simulink model "TST_InjCrv_PoI2Cor"  (R2016b)
settings: Solver=FixedStepDiscrete  StartTime=0.0  StopTime=simTime  FixedStep=sampleTime  RelTol=1e-3
values from neighbouring files (symbols this model uses):
  testCase = 1    [initTST_InjCrv_PoI2Cor_001.m]
libraries: simulink x5, UnitTest_Lib x3
settings Model: Creator=zhengjinyan  LastModifiedBy=zhengjinyan
settings DebuggingCC: SignalRangeChecking=error

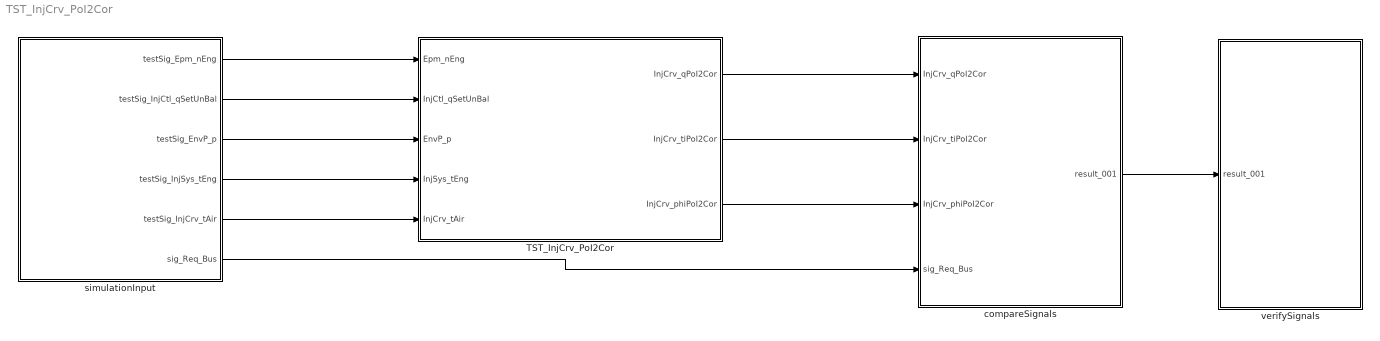
== system TST_InjCrv_PoI2Cor ==
  TST_InjCrv_PoI2Cor : Subsystem
  compareSignals : Subsystem
  simulationInput : Subsystem
  verifySignals : Subsystem
  wires:
  simulationInput/1(testSig_Epm_nEng) -> TST_InjCrv_PoI2Cor/1(Epm_nEng)
  simulationInput/2(testSig_InjCtl_qSetUnBal) -> TST_InjCrv_PoI2Cor/2(InjCtl_qSetUnBal)
  simulationInput/3(testSig_EnvP_p) -> TST_InjCrv_PoI2Cor/3(EnvP_p)
  simulationInput/4(testSig_InjSys_tEng) -> TST_InjCrv_PoI2Cor/4(InjSys_tEng)
  simulationInput/5(testSig_InjCrv_tAir) -> TST_InjCrv_PoI2Cor/5(InjCrv_tAir)
  TST_InjCrv_PoI2Cor/1(InjCrv_qPoI2Cor) -> compareSignals/1(InjCrv_qPoI2Cor)
  TST_InjCrv_PoI2Cor/2(InjCrv_tiPoI2Cor) -> compareSignals/2(InjCrv_tiPoI2Cor)
  TST_InjCrv_PoI2Cor/3(InjCrv_phiPoI2Cor) -> compareSignals/3(InjCrv_phiPoI2Cor)
  simulationInput/6(sig_Req_Bus) -> compareSignals/4(sig_Req_Bus)
  compareSignals/1(result_001) -> verifySignals/1(result_001)

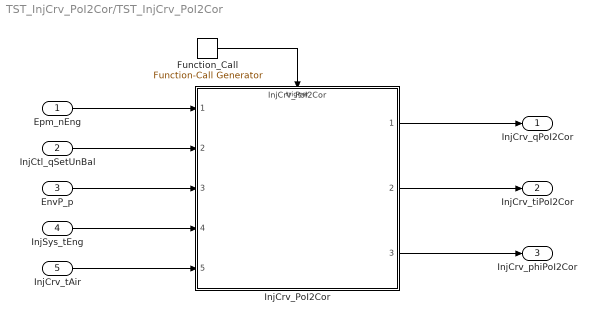
== system TST_InjCrv_PoI2Cor/TST_InjCrv_PoI2Cor ==
  Epm_nEng : Inport
  InjCtl_qSetUnBal : Inport  Port=2
  EnvP_p : Inport  Port=3
  InjSys_tEng : Inport  Port=4
  InjCrv_tAir : Inport  Port=5
  Function_Call : simulink/Ports & Subsystems/Function-Call Generator  sample_time=sampleTime  numberOfIterations=1
  InjCrv_PoI2Cor : ModelReference  ModelNameDialog=InjCrv_PoI2Cor  SimulationMode=Normal  ModelReferenceVersion=1.32  TriggerPortName=function  TriggerPortTriggerType=function-call  TriggerPortStatesWhenEnabling=held
  InjCrv_qPoI2Cor : Outport
  InjCrv_tiPoI2Cor : Outport  Port=2
  InjCrv_phiPoI2Cor : Outport  Port=3
  wires:
  Function_Call/1 -> InjCrv_PoI2Cor/Trigger
  Epm_nEng/1 -> InjCrv_PoI2Cor/1
  InjCtl_qSetUnBal/1 -> InjCrv_PoI2Cor/2
  EnvP_p/1 -> InjCrv_PoI2Cor/3
  InjSys_tEng/1 -> InjCrv_PoI2Cor/4
  InjCrv_tAir/1 -> InjCrv_PoI2Cor/5
  InjCrv_PoI2Cor/1 -> InjCrv_qPoI2Cor/1
  InjCrv_PoI2Cor/2 -> InjCrv_tiPoI2Cor/1
  InjCrv_PoI2Cor/3 -> InjCrv_phiPoI2Cor/1

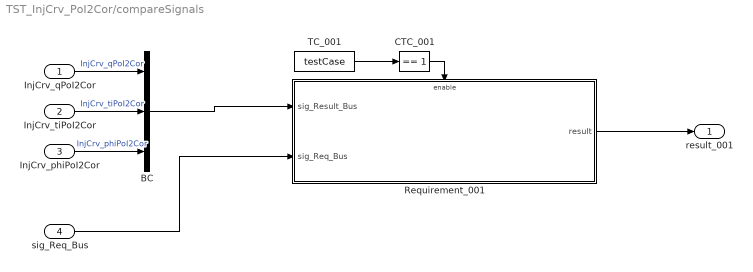
== system TST_InjCrv_PoI2Cor/compareSignals ==
  InjCrv_qPoI2Cor : Inport
  InjCrv_tiPoI2Cor : Inport  Port=2
  InjCrv_phiPoI2Cor : Inport  Port=3
  sig_Req_Bus : Inport  Port=4
  BC : BusCreator  Inputs=3
  CTC_001 : simulink/Logic and Bit Operations/Compare To Constant  relop===  const=1  OutDataTypeStr=boolean
  Requirement_001 : Subsystem
  TC_001 : Constant  Value=testCase
  result_001 : Outport
  wires:
  InjCrv_qPoI2Cor/1 -> BC/1  "InjCrv_qPoI2Cor"
  InjCrv_tiPoI2Cor/1 -> BC/2  "InjCrv_tiPoI2Cor"
  InjCrv_phiPoI2Cor/1 -> BC/3  "InjCrv_phiPoI2Cor"
  TC_001/1 -> CTC_001/1
  CTC_001/1 -> Requirement_001/Enable
  sig_Req_Bus/1 -> Requirement_001/2(sig_Req_Bus)
  BC/1 -> Requirement_001/1(sig_Result_Bus)
  Requirement_001/1(result) -> result_001/1

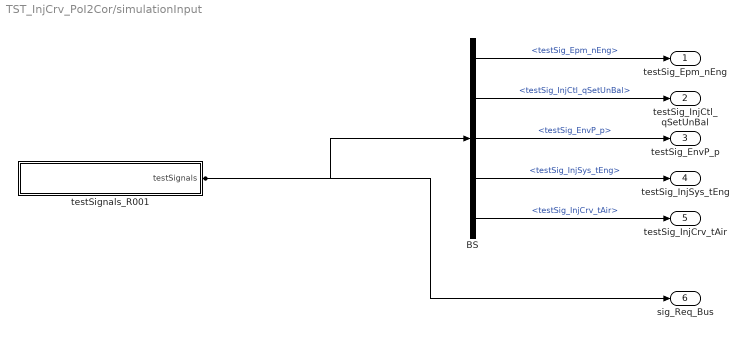
== system TST_InjCrv_PoI2Cor/simulationInput ==
  BS : BusSelector  OutputSignals=testSig_Epm_nEng,testSig_InjCtl_qSetUnBal,testSig_EnvP_p,testSig_InjSys_tEng,testSig_InjCrv_tAir
  testSignals_R001 : Subsystem
  testSig_Epm_nEng : Outport
  testSig_InjCtl_qSetUnBal : Outport  Port=2
  testSig_EnvP_p : Outport  Port=3
  testSig_InjSys_tEng : Outport  Port=4
  testSig_InjCrv_tAir : Outport  Port=5
  sig_Req_Bus : Outport  Port=6
  wires:
  BS/1 -> testSig_Epm_nEng/1  "<testSig_Epm_nEng>"
  BS/2 -> testSig_InjCtl_qSetUnBal/1  "<testSig_InjCtl_qSetUnBal>"
  BS/3 -> testSig_EnvP_p/1  "<testSig_EnvP_p>"
  BS/4 -> testSig_InjSys_tEng/1  "<testSig_InjSys_tEng>"
  BS/5 -> testSig_InjCrv_tAir/1  "<testSig_InjCrv_tAir>"
  testSignals_R001/1(testSignals) -> BS/1, sig_Req_Bus/1

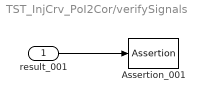
== system TST_InjCrv_PoI2Cor/verifySignals ==
  result_001 : Inport
  Assertion_001 : Assertion  Enabled=off
  wires:
  result_001/1 -> Assertion_001/1

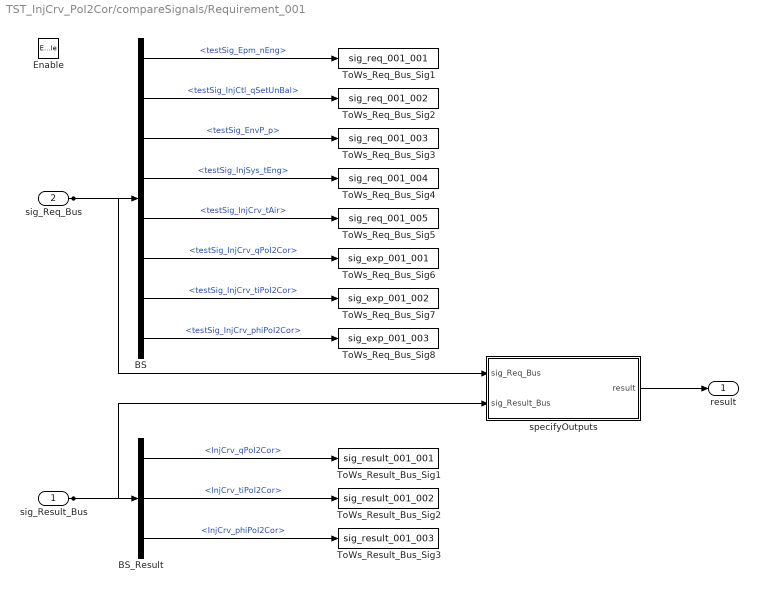
== system TST_InjCrv_PoI2Cor/compareSignals/Requirement_001 ==
  sig_Result_Bus : Inport
  sig_Req_Bus : Inport  Port=2
  Enable : EnablePort
  BS : BusSelector  OutputSignals=testSig_Epm_nEng,testSig_InjCtl_qSetUnBal,testSig_EnvP_p,testSig_InjSys_tEng,testSig_InjCrv_tAir,testSig_InjCrv_qPoI2Cor,testSig_InjCrv_tiPoI2Cor,testSig_InjCrv_phiPoI2Cor
  BS_Result : BusSelector  OutputSignals=InjCrv_qPoI2Cor,InjCrv_tiPoI2Cor,InjCrv_phiPoI2Cor
  ToWs_Req_Bus_Sig1 : ToWorkspace  VariableName=sig_req_001_001  SaveFormat=Structure With Time
  ToWs_Req_Bus_Sig2 : ToWorkspace  VariableName=sig_req_001_002  SaveFormat=Structure With Time
  ToWs_Req_Bus_Sig3 : ToWorkspace  VariableName=sig_req_001_003  SaveFormat=Structure With Time
  ToWs_Req_Bus_Sig4 : ToWorkspace  VariableName=sig_req_001_004  SaveFormat=Structure With Time
  ToWs_Req_Bus_Sig5 : ToWorkspace  VariableName=sig_req_001_005  SaveFormat=Structure With Time
  ToWs_Req_Bus_Sig6 : ToWorkspace  VariableName=sig_exp_001_001  SaveFormat=Structure With Time
  ToWs_Req_Bus_Sig7 : ToWorkspace  VariableName=sig_exp_001_002  SaveFormat=Structure With Time
  ToWs_Req_Bus_Sig8 : ToWorkspace  VariableName=sig_exp_001_003  SaveFormat=Structure With Time
  ToWs_Result_Bus_Sig1 : ToWorkspace  VariableName=sig_result_001_001  SaveFormat=Structure With Time
  ToWs_Result_Bus_Sig2 : ToWorkspace  VariableName=sig_result_001_002  SaveFormat=Structure With Time
  ToWs_Result_Bus_Sig3 : ToWorkspace  VariableName=sig_result_001_003  SaveFormat=Structure With Time
  specifyOutputs : Subsystem
  result : Outport
  wires:
  sig_Req_Bus/1 -> BS/1, specifyOutputs/1(sig_Req_Bus)
  BS/1 -> ToWs_Req_Bus_Sig1/1  "<testSig_Epm_nEng>"
  BS/2 -> ToWs_Req_Bus_Sig2/1  "<testSig_InjCtl_qSetUnBal>"
  BS/3 -> ToWs_Req_Bus_Sig3/1  "<testSig_EnvP_p>"
  BS/4 -> ToWs_Req_Bus_Sig4/1  "<testSig_InjSys_tEng>"
  BS/5 -> ToWs_Req_Bus_Sig5/1  "<testSig_InjCrv_tAir>"
  BS/6 -> ToWs_Req_Bus_Sig6/1  "<testSig_InjCrv_qPoI2Cor>"
  BS/7 -> ToWs_Req_Bus_Sig7/1  "<testSig_InjCrv_tiPoI2Cor>"
  BS/8 -> ToWs_Req_Bus_Sig8/1  "<testSig_InjCrv_phiPoI2Cor>"
  sig_Result_Bus/1 -> BS_Result/1, specifyOutputs/2(sig_Result_Bus)
  BS_Result/1 -> ToWs_Result_Bus_Sig1/1  "<InjCrv_qPoI2Cor>"
  BS_Result/2 -> ToWs_Result_Bus_Sig2/1  "<InjCrv_tiPoI2Cor>"
  BS_Result/3 -> ToWs_Result_Bus_Sig3/1  "<InjCrv_phiPoI2Cor>"
  specifyOutputs/1(result) -> result/1

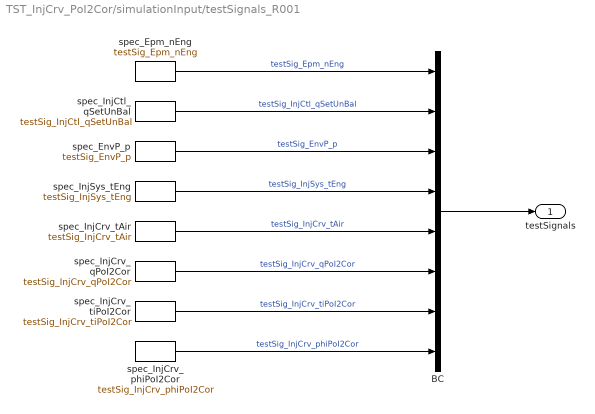
== system TST_InjCrv_PoI2Cor/simulationInput/testSignals_R001 ==
  BC : BusCreator  Inputs=8
  spec_EnvP_p : FromWorkspace  VariableName=testSig_EnvP_p  Interpolate=off  OutputAfterFinalValue=Holding final value
  spec_Epm_nEng : FromWorkspace  VariableName=testSig_Epm_nEng  Interpolate=off  OutputAfterFinalValue=Holding final value
  spec_InjCrv_phiPoI2Cor : FromWorkspace  VariableName=testSig_InjCrv_phiPoI2Cor  Interpolate=off  OutputAfterFinalValue=Holding final value
  spec_InjCrv_qPoI2Cor : FromWorkspace  VariableName=testSig_InjCrv_qPoI2Cor  Interpolate=off  OutputAfterFinalValue=Holding final value
  spec_InjCrv_tAir : FromWorkspace  VariableName=testSig_InjCrv_tAir  Interpolate=off  OutputAfterFinalValue=Holding final value
  spec_InjCrv_tiPoI2Cor : FromWorkspace  VariableName=testSig_InjCrv_tiPoI2Cor  Interpolate=off  OutputAfterFinalValue=Holding final value
  spec_InjCtl_qSetUnBal : FromWorkspace  VariableName=testSig_InjCtl_qSetUnBal  Interpolate=off  OutputAfterFinalValue=Holding final value
  spec_InjSys_tEng : FromWorkspace  VariableName=testSig_InjSys_tEng  Interpolate=off  OutputAfterFinalValue=Holding final value
  testSignals : Outport
  wires:
  BC/1 -> testSignals/1
  spec_Epm_nEng/1 -> BC/1  "testSig_Epm_nEng"
  spec_InjCtl_qSetUnBal/1 -> BC/2  "testSig_InjCtl_qSetUnBal"
  spec_EnvP_p/1 -> BC/3  "testSig_EnvP_p"
  spec_InjSys_tEng/1 -> BC/4  "testSig_InjSys_tEng"
  spec_InjCrv_tAir/1 -> BC/5  "testSig_InjCrv_tAir"
  spec_InjCrv_qPoI2Cor/1 -> BC/6  "testSig_InjCrv_qPoI2Cor"
  spec_InjCrv_tiPoI2Cor/1 -> BC/7  "testSig_InjCrv_tiPoI2Cor"
  spec_InjCrv_phiPoI2Cor/1 -> BC/8  "testSig_InjCrv_phiPoI2Cor"

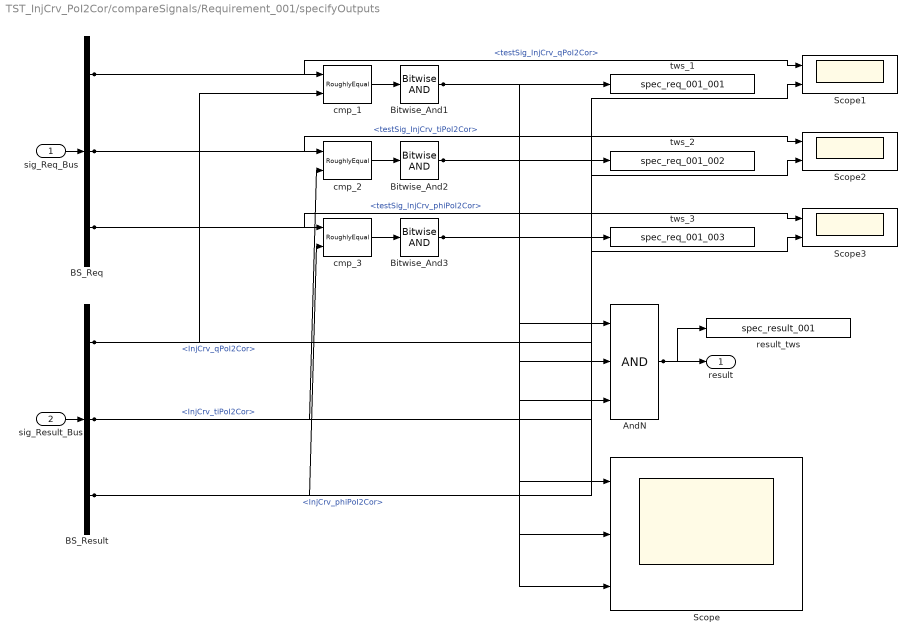
== system TST_InjCrv_PoI2Cor/compareSignals/Requirement_001/specifyOutputs ==
  sig_Req_Bus : Inport
  sig_Result_Bus : Inport  Port=2
  AndN : Logic  Inputs=3
  BS_Req : BusSelector  OutputSignals=testSig_InjCrv_qPoI2Cor,testSig_InjCrv_tiPoI2Cor,testSig_InjCrv_phiPoI2Cor
  BS_Result : BusSelector  OutputSignals=InjCrv_qPoI2Cor,InjCrv_tiPoI2Cor,InjCrv_phiPoI2Cor
  Bitwise_And1 : simulink/Logic and Bit Operations/Bitwise Operator  logicop=AND  UseBitMask=off  BitMask=bin2dec('11011001')  BitMaskRealWorld=Stored Integer
  Bitwise_And2 : simulink/Logic and Bit Operations/Bitwise Operator  logicop=AND  UseBitMask=off  BitMask=bin2dec('11011001')  BitMaskRealWorld=Stored Integer
  Bitwise_And3 : simulink/Logic and Bit Operations/Bitwise Operator  logicop=AND  UseBitMask=off  BitMask=bin2dec('11011001')  BitMaskRealWorld=Stored Integer
  Scope : Scope  NumInputPorts=3
  Scope1 : Scope  NumInputPorts=2
  Scope2 : Scope  NumInputPorts=2
  Scope3 : Scope  NumInputPorts=2
  cmp_1 : UnitTest_Lib/RoughlyEqual  slope=0.1
  cmp_2 : UnitTest_Lib/RoughlyEqual  slope=0.1
  cmp_3 : UnitTest_Lib/RoughlyEqual  slope=0.1
  result_tws : ToWorkspace  VariableName=spec_result_001
  tws_1 : ToWorkspace  VariableName=spec_req_001_001
  tws_2 : ToWorkspace  VariableName=spec_req_001_002
  tws_3 : ToWorkspace  VariableName=spec_req_001_003
  result : Outport
  wires:
  sig_Req_Bus/1 -> BS_Req/1
  sig_Result_Bus/1 -> BS_Result/1
  AndN/1 -> result/1, result_tws/1
  BS_Req/1 -> cmp_1/1, Scope1/1  "<testSig_InjCrv_qPoI2Cor>"
  BS_Result/1 -> cmp_1/2, Scope1/2  "<InjCrv_qPoI2Cor>"
  cmp_1/1 -> Bitwise_And1/1
  Bitwise_And1/1 -> tws_1/1, AndN/1, Scope/1
  BS_Req/2 -> cmp_2/1, Scope2/1  "<testSig_InjCrv_tiPoI2Cor>"
  BS_Result/2 -> cmp_2/2, Scope2/2  "<InjCrv_tiPoI2Cor>"
  cmp_2/1 -> Bitwise_And2/1
  Bitwise_And2/1 -> tws_2/1, AndN/2, Scope/2
  BS_Req/3 -> cmp_3/1, Scope3/1  "<testSig_InjCrv_phiPoI2Cor>"
  BS_Result/3 -> cmp_3/2, Scope3/2  "<InjCrv_phiPoI2Cor>"
  cmp_3/1 -> Bitwise_And3/1
  Bitwise_And3/1 -> tws_3/1, AndN/3, Scope/3
